simulink model "rx"  (R2012b)
settings: Solver=ode45  StartTime=0.0  StopTime=10.0  RelTol=1e-3
undefined symbols (not defined in the file or in its folder): gcbh, xlBlockLoadCallback, xlGetNormalizedPeriod
libraries: xbsIndex_r4 x88, xbsEDKLib_r4 x1
(part 3 of 3)

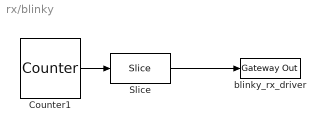
== system rx/blinky ==
  Counter1 : xbsIndex_r4/Counter  cnt_type=Free Running  cnt_to=Inf  operation=Up  start_count=0  cnt_by_val=1  arith_type=Unsigned  n_bits=25  bin_pt=0  load_pin=off  rst=off  en=off  explicit_period=on  period=1  dbl_ovrd=off  use_behavioral_HDL=off  implementation=Fabric  block_type=counter
  Slice : xbsIndex_r4/Slice  nbits=1  boolean_output=off  mode=Upper Bit Location + Width  bit1=0  base1=MSB of Input  bit0=0  base0=LSB of Input  dbl_ovrd=off  block_type=slice
  blinky_rx_driver : xbsIndex_r4/Gateway Out  inherit_from_input=off  hdl_port=on  timing_constraint=None  locs_specified=off  LOCs={}  UseAsDAC=off  DACChannel='1'  block_type=gatewayout
  wires:
  Counter1/1 -> Slice/1
  Slice/1 -> blinky_rx_driver/1

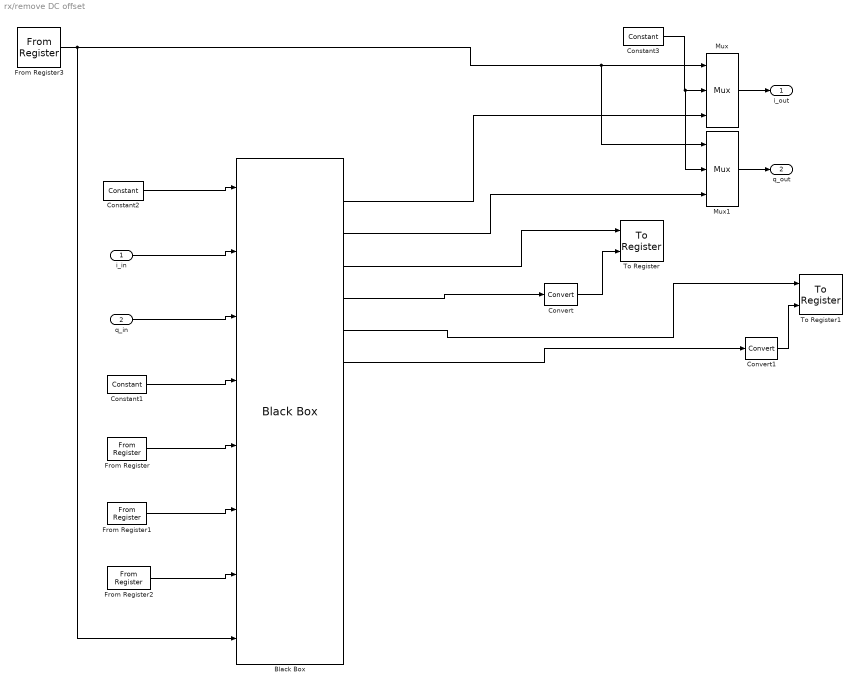
== system rx/remove DC offset ==
  i_in : Inport
  q_in : Inport  Port=2
  Black Box : xbsIndex_r4/Black Box  init_code=dc_offset_correction_FixPt_xsgbbxcfg  sim_method=Inactive  verbose=off  block_type=blackbox2
  Constant1 : xbsIndex_r4/Constant  const=1  gui_display_data_type=Fixed-point  arith_type=Unsigned  n_bits=12  bin_pt=0  preci_type=Single  exp_width=8  frac_width=24  explicit_period=on  period=1  equ=P=C  opselect=C  inp2=PCIN>>17  opr=+  inp1=P  carry=CIN  dbl_ovrd=off  block_type=constant
  Constant2 : xbsIndex_r4/Constant  const=0  gui_display_data_type=Fixed-point  arith_type=Unsigned  n_bits=1  bin_pt=0  preci_type=Single  exp_width=8  frac_width=24  explicit_period=on  period=1  equ=P=C  opselect=C  inp2=PCIN>>17  opr=+  inp1=P  carry=CIN  dbl_ovrd=off  block_type=constant
  Constant3 : xbsIndex_r4/Constant  const=0  gui_display_data_type=Fixed-point  arith_type=Signed (2's comp)  n_bits=12  bin_pt=0  preci_type=Single  exp_width=8  frac_width=24  explicit_period=on  period=1  equ=P=C  opselect=C  inp2=PCIN>>17  opr=+  inp1=P  carry=CIN  dbl_ovrd=off  block_type=constant
  Convert : xbsIndex_r4/Convert  gui_display_data_type=Boolean  arith_type=Boolean  n_bits=16  bin_pt=14  float_type=Single  exp_bits=8  fraction_bits=24  quantization=Truncate  overflow=Wrap  en=off  latency=0  dbl_ovrd=off  pipeline=off  block_type=convert
  Convert1 : xbsIndex_r4/Convert  gui_display_data_type=Boolean  arith_type=Boolean  n_bits=16  bin_pt=14  float_type=Single  exp_bits=8  fraction_bits=24  quantization=Truncate  overflow=Wrap  en=off  latency=0  dbl_ovrd=off  pipeline=off  block_type=convert
  From Register : xbsIndex_r4/From Register  shared_memory_name='agc_en'  init=0  period=1  ownership=Owned and initialized elsewhere  gui_display_data_type=Fixed-point  arith_type=Unsigned  n_bits=1  bin_pt=0  preci_type=Single  dbl_ovrd=off  block_type=fromreg
      settings: AttributesFormatString=<< %<shared_memory_name> >>  infoedit="Register block that reads data to a shared memory register.  Delay of one sample period."
  From Register1 : xbsIndex_r4/From Register  shared_memory_name='rssi_low_goal'  init=0  period=1  ownership=Owned and initialized elsewhere  gui_display_data_type=Fixed-point  arith_type=Unsigned  n_bits=24  bin_pt=0  preci_type=Single  dbl_ovrd=off  block_type=fromreg
      settings: AttributesFormatString=<< %<shared_memory_name> >>  infoedit="Register block that reads data to a shared memory register.  Delay of one sample period."
  From Register2 : xbsIndex_r4/From Register  shared_memory_name='rssi_high_goal'  init=0  period=1  ownership=Owned and initialized elsewhere  gui_display_data_type=Fixed-point  arith_type=Unsigned  n_bits=24  bin_pt=0  preci_type=Single  dbl_ovrd=off  block_type=fromreg
      settings: AttributesFormatString=<< %<shared_memory_name> >>  infoedit="Register block that reads data to a shared memory register.  Delay of one sample period."
  From Register3 : xbsIndex_r4/From Register  shared_memory_name='rx_en'  init=0  period=1  ownership=Owned and initialized elsewhere  gui_display_data_type=Fixed-point  arith_type=Unsigned  n_bits=1  bin_pt=0  preci_type=Single  dbl_ovrd=off  block_type=fromreg
      settings: AttributesFormatString=<< %<shared_memory_name> >>  infoedit="Register block that reads data to a shared memory register.  Delay of one sample period."
  Mux : xbsIndex_r4/Mux  inputs=2  en=off  latency=0  precision=Full  arith_type=Unsigned  n_bits=16  bin_pt=14  quantization=Truncate  overflow=Wrap  dbl_ovrd=off  block_type=mux
  Mux1 : xbsIndex_r4/Mux  inputs=2  en=off  latency=0  precision=Full  arith_type=Unsigned  n_bits=16  bin_pt=14  quantization=Truncate  overflow=Wrap  dbl_ovrd=off  block_type=mux
  To Register : xbsIndex_r4/To Register  shared_memory_name='rssi'  init=0  ownership=Locally owned and initialized  explicit_data_type=on  gui_display_data_type=Fixed-point  arith_type=Unsigned  n_bits=24  bin_pt=0  preci_type=Single  dbl_ovrd=off  block_type=toreg
      settings: AttributesFormatString=<< %<shared_memory_name> >>  infoedit="Register block that writes data to a shared memory register.  Delay of one sample period."
  To Register1 : xbsIndex_r4/To Register  shared_memory_name='dir'  init=0  ownership=Locally owned and initialized  explicit_data_type=on  gui_display_data_type=Fixed-point  arith_type=Unsigned  n_bits=2  bin_pt=0  preci_type=Single  dbl_ovrd=off  block_type=toreg
      settings: AttributesFormatString=<< %<shared_memory_name> >>  infoedit="Register block that writes data to a shared memory register.  Delay of one sample period."
  i_out : Outport
  q_out : Outport  Port=2
  wires:
  Constant2/1 -> Black Box/1
  q_in/1 -> Black Box/3
  Constant1/1 -> Black Box/4
  Black Box/5 -> Convert/1
  Convert/1 -> To Register/2
  Black Box/4 -> To Register/1
  From Register/1 -> Black Box/5
  From Register1/1 -> Black Box/6
  From Register2/1 -> Black Box/7
  Black Box/7 -> Convert1/1
  Convert1/1 -> To Register1/2
  Black Box/6 -> To Register1/1
  i_in/1 -> Black Box/2
  From Register3/1 -> Black Box/8, Mux1/1, Mux/1
  Constant3/1 -> Mux1/2, Mux/2
  Black Box/2 -> Mux/3
  Mux/1 -> i_out/1
  Mux1/1 -> q_out/1
  Black Box/3 -> Mux1/3

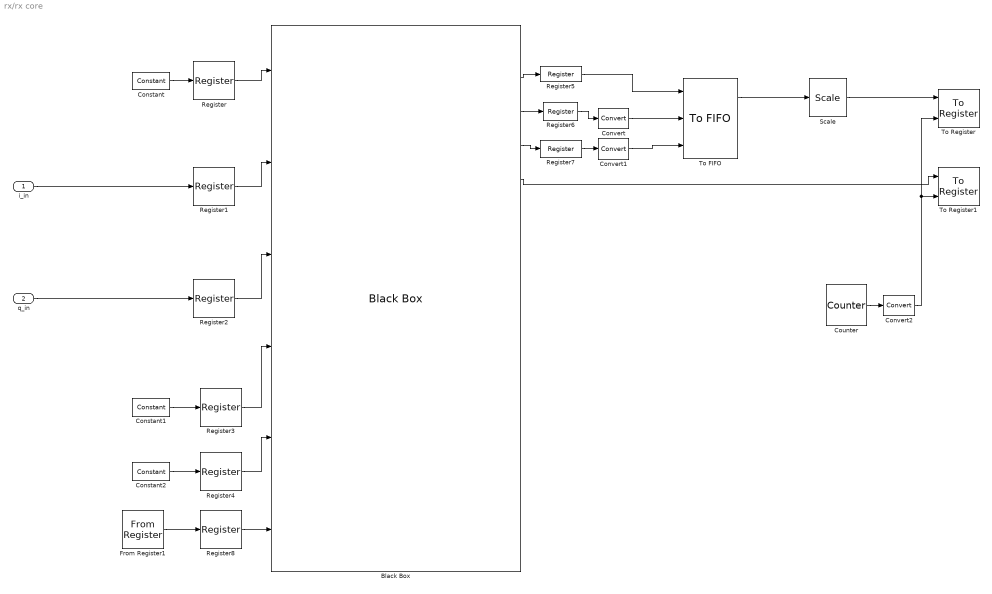
== system rx/rx core ==
  i_in : Inport
  q_in : Inport  Port=2
  Black Box : xbsIndex_r4/Black Box  init_code=qpsk_rx_FixPt_xsgbbxcfg  sim_method=Inactive  verbose=off  block_type=blackbox2
  Constant : xbsIndex_r4/Constant  const=0  gui_display_data_type=Fixed-point  arith_type=Unsigned  n_bits=1  bin_pt=0  preci_type=Single  exp_width=8  frac_width=24  explicit_period=on  period=1  equ=P=C  opselect=C  inp2=PCIN>>17  opr=+  inp1=P  carry=CIN  dbl_ovrd=off  block_type=constant
  Constant1 : xbsIndex_r4/Constant  const=floor(.01*2^12)  gui_display_data_type=Fixed-point  arith_type=Unsigned  n_bits=12  bin_pt=0  preci_type=Single  exp_width=8  frac_width=24  explicit_period=on  period=1  equ=P=C  opselect=C  inp2=PCIN>>17  opr=+  inp1=P  carry=CIN  dbl_ovrd=off  block_type=constant
  Constant2 : xbsIndex_r4/Constant  const=floor(.01*8*2^12)  gui_display_data_type=Fixed-point  arith_type=Unsigned  n_bits=12  bin_pt=0  preci_type=Single  exp_width=8  frac_width=24  explicit_period=on  period=1  equ=P=C  opselect=C  inp2=PCIN>>17  opr=+  inp1=P  carry=CIN  dbl_ovrd=off  block_type=constant
  Convert : xbsIndex_r4/Convert  gui_display_data_type=Boolean  arith_type=Boolean  n_bits=16  bin_pt=14  float_type=Single  exp_bits=8  fraction_bits=24  quantization=Truncate  overflow=Wrap  en=off  latency=0  dbl_ovrd=off  pipeline=off  block_type=convert
  Convert1 : xbsIndex_r4/Convert  gui_display_data_type=Boolean  arith_type=Boolean  n_bits=16  bin_pt=14  float_type=Single  exp_bits=8  fraction_bits=24  quantization=Truncate  overflow=Wrap  en=off  latency=0  dbl_ovrd=off  pipeline=off  block_type=convert
  Convert2 : xbsIndex_r4/Convert  gui_display_data_type=Boolean  arith_type=Boolean  n_bits=16  bin_pt=14  float_type=Single  exp_bits=8  fraction_bits=24  quantization=Truncate  overflow=Wrap  en=off  latency=0  dbl_ovrd=off  pipeline=off  block_type=convert
  Counter : xbsIndex_r4/Counter  cnt_type=Free Running  cnt_to=Inf  operation=Up  start_count=0  cnt_by_val=1  arith_type=Unsigned  n_bits=1  bin_pt=0  load_pin=off  rst=off  en=off  explicit_period=on  period=1  dbl_ovrd=off  use_behavioral_HDL=off  implementation=Fabric  block_type=counter
  From Register1 : xbsIndex_r4/From Register  shared_memory_name='mcu_rx_ready'  init=0  period=1  ownership=Owned and initialized elsewhere  gui_display_data_type=Fixed-point  arith_type=Unsigned  n_bits=1  bin_pt=0  preci_type=Single  dbl_ovrd=off  block_type=fromreg
      settings: AttributesFormatString=<< %<shared_memory_name> >>  infoedit="Register block that reads data to a shared memory register.  Delay of one sample period."
  Register{,1..8} (9 alike) : xbsIndex_r4/Register  init=0  rst=off  en=off  dbl_ovrd=off  block_type=register
  Scale : xbsIndex_r4/Scale  scale_factor=10  dbl_ovrd=off  block_type=scale
  To FIFO : xbsIndex_r4/To FIFO  shared_memory_name='rx_fifo'  ownership=Locally owned  mem_type=Block RAM  performance_options=Standard_FIFO  infoedit1=Available only for V4, V5, V6, V7, K7, A7 and Zynq devices.  embedded_registers=off  depth=1K  percent_nbits=10  has_arst=on  use_percent_full_port=on  explicit_data_type=on  gui_display_data_type=Fixed-point  arith_type=Unsigned  n_bits=8  bin_pt=0  preci_type=Single  dbl_ovrd=off  block_type=tofifo
      settings: AttributesFormatString=<< %<shared_memory_name> >>  infoedit=First-in-first-out (FIFO) block that writes FIFO data to shared memory storage.
  To Register : xbsIndex_r4/To Register  shared_memory_name='percent_full'  init=0  ownership=Locally owned and initialized  explicit_data_type=on  gui_display_data_type=Fixed-point  arith_type=Unsigned  n_bits=10  bin_pt=0  preci_type=Single  dbl_ovrd=off  block_type=toreg
      settings: AttributesFormatString=<< %<shared_memory_name> >>  infoedit="Register block that writes data to a shared memory register.  Delay of one sample period."
  To Register1 : xbsIndex_r4/To Register  shared_memory_name='num_bytes_ready'  init=0  ownership=Locally owned and initialized  explicit_data_type=on  gui_display_data_type=Fixed-point  arith_type=Unsigned  n_bits=9  bin_pt=0  preci_type=Single  dbl_ovrd=off  block_type=toreg
      settings: AttributesFormatString=<< %<shared_memory_name> >>  infoedit="Register block that writes data to a shared memory register.  Delay of one sample period."
  wires:
  Black Box/3 -> Register6/1
  Black Box/4 -> Register7/1
  Convert/1 -> To FIFO/2
  Register/1 -> Black Box/1
  Register2/1 -> Black Box/3
  Register3/1 -> Black Box/4
  Register4/1 -> Black Box/5
  Register5/1 -> To FIFO/1
  Register6/1 -> Convert/1
  Register1/1 -> Black Box/2
  Constant/1 -> Register/1
  Constant1/1 -> Register3/1
  Constant2/1 -> Register4/1
  Black Box/2 -> Register5/1
  Register7/1 -> Convert1/1
  Convert1/1 -> To FIFO/3
  To FIFO/1 -> Scale/1
  Register8/1 -> Black Box/6
  From Register1/1 -> Register8/1
  Counter/1 -> Convert2/1
  Convert2/1 -> To Register1/2, To Register/2
  Scale/1 -> To Register/1
  q_in/1 -> Register2/1
  Black Box/5 -> To Register1/1
  i_in/1 -> Register1/1
